simulink model "insulin_model"  (R2024b)
settings: Solver=ode15s  StartTime=0.0  StopTime=86400  MaxStep=0.5  RelTol=1e-3
libraries: fl_lib x11, nesl_utility x4, eeGeneralControl x1, SimscapeFluids_lib x1
settings Model: Creator=14083  LastModifiedBy=14083

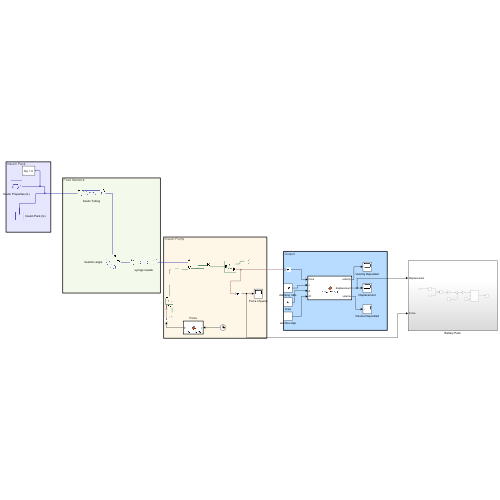
[thumbnail: Simulink's stored preview of the top-level diagram]
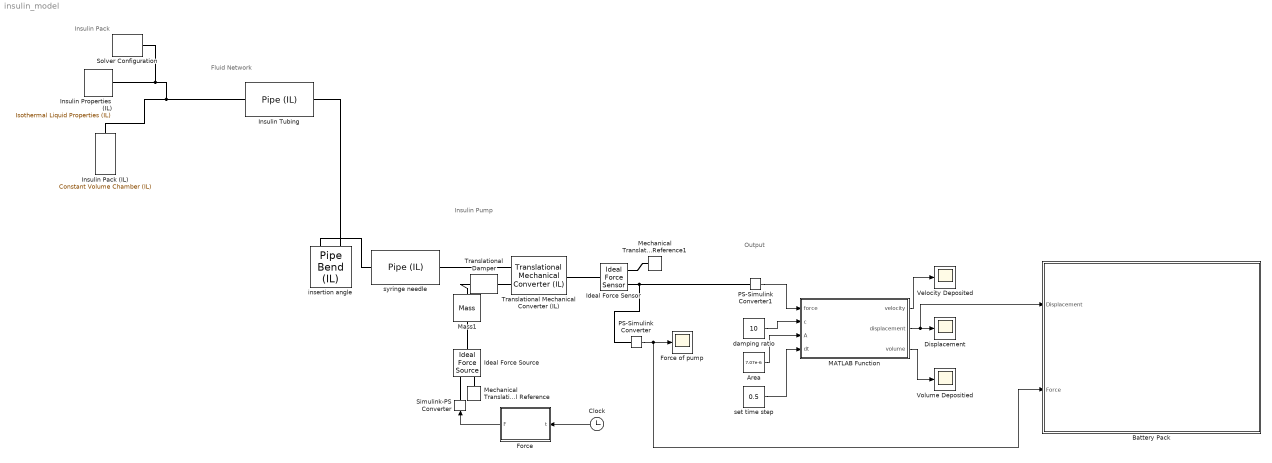
== system insulin_model ==
  note: Fluid Network
  note: Output
  note: Insulin Pump
  note: Insulin Pack
  Area : Constant  Value=7.07e-6
  Battery Pack : Subsystem
  Clock : Clock
  Displacement : Scope
  Force : MATLAB Function  TreatAsAtomicUnit=on
  Force of pump : Scope
  Ideal Force Sensor : fl_lib/Mechanical/Mechanical Sensors/Ideal Force Sensor
  Ideal Force Source : fl_lib/Mechanical/Mechanical Sources/Ideal Force Source
  Insulin Pack (IL) : fl_lib/Isothermal Liquid/Elements/Constant Volume Chamber (IL)  volume=0.00068 l  p_I_specify=off  p_I_priority=High  p_I=0.101325 MPa  p_I_nominal_specify=off  p_I_nominal_value=1  p_I_nominal_unit=MPa
      settings: InternalSimscapePortConfiguration="{\"Bottom\":[],\"Left\":[{\"id\":\"A\",\"label\":\"A\",\"type\":\"foundation.isothermal_liquid.isothermal_liquid\"}],\"Right\":[],\"Top\":[]}"
  Insulin Properties (IL) : fl_lib/Isothermal Liquid/Utilities/Isothermal Liquid Properties (IL)  rho_L_atm=998.2 kg/m^3  bulk_modulus_model=foundation.enum.bulk_modulus_model.const  beta_gain=6  beta_L_atm=2.1791e9 Pa  nu_atm=1.0034e-6 m^2/s  p_atm=0.101325 MPa  p_min=1 Pa  properties_range_check=simscape.enum.assert.action.error  air_fraction=0.005  polytropic_index=1.0  rho_g_atm=1.225 kg/m^3  air_dissolution_model=false  p_crit=3 MPa
  Insulin Tubing : fl_lib/Isothermal Liquid/Elements/Pipe (IL)  length=23 in  area=(1.5^2)*pi/4 mm^2  Dh=1.5 mm  length_add=1 m  roughness=15e-6 m  Re_lam=2000  Re_tur=4000  shape_factor=64  dynamic_compressibility=true  inertia=false  p0=0.101325 MPa  mdot0=0 kg/s
      settings: InternalSimscapePortConfiguration="{\"Bottom\":[],\"Left\":[{\"id\":\"A\",\"label\":\"A\",\"type\":\"foundation.isothermal_liquid.isothermal_liquid\"}],\"Right\":[{\"id\":\"B\",\"label\":\"B\",\"type\":\"foundation.isothermal_liquid.isothermal_liquid\"}],\"Top\":[]}"
  MATLAB Function : MATLAB Function  TreatAsAtomicUnit=on  SystemSampleTime=0.5
  Mass1 : fl_lib/Mechanical/Translational Elements/Mass  mass=0.01 kg  num_ports=foundation.enum.numPorts2.two  v_specify=off  v_priority=High  v=0 m/s  v_nominal_specify=off  v_nominal_value=1  v_nominal_unit=m/s  f_specify=off  f_priority=None  f=0 N  f_nominal_specify=off  f_nominal_value=1  f_nominal_unit=N
      settings: InternalSimscapePortConfiguration="{\"Bottom\":[],\"Left\":[{\"id\":\"M\",\"label\":\"\",\"type\":\"foundation.mechanical.translational.translational\"}],\"Right\":[{\"id\":\"N\",\"label\":\"\",\"type\":\"foundation.mechanical.translational.translational\"}],\"Top\":[]}"
  Mechanical Translational Reference : fl_lib/Mechanical/Translational Elements/Mechanical Translational Reference
  Mechanical Translational Reference1 : fl_lib/Mechanical/Translational Elements/Mechanical Translational Reference
  PS-Simulink Converter : nesl_utility/PS-Simulink Converter  PhysicalDomain=network_engine_domain  SubClassName=ps_output  LeftPortType=input  RightPortType=output  PseudoPeriodic=off  Frequencies=[]  VectorFormat=inherit  Unit=inherit  AffineConversion=off
  PS-Simulink Converter1 : nesl_utility/PS-Simulink Converter  PhysicalDomain=network_engine_domain  SubClassName=ps_output  LeftPortType=input  RightPortType=output  PseudoPeriodic=off  Frequencies=[]  VectorFormat=inherit  Unit=inherit  AffineConversion=off
  Simulink-PS Converter : nesl_utility/Simulink-PS Converter  PhysicalDomain=network_engine_domain  SubClassName=ps_input  LeftPortType=input  RightPortType=output  PseudoPeriodic=off  Frequencies=[]  NoiseDistribution=none  NoiseParameters=[]  Unit=1  AffineConversion=off  FilteringAndDerivatives=provide  SimscapeFilterOrder=1  InputFilterTimeConstant=0.001  UdotUserProvided=0
  Solver Configuration : nesl_utility/Solver Configuration  PhysicalDomain=network_engine_domain  SubClassName=solver  LeftPortType=input  RightPortType=generic  Tones=[]  Harmonics=[]  SimulateNoise=off  Profile=off  UseLocalSampling=off  EnableSwitchedLinearOptims=on  FrequencyDomain=off  UseCCode=off  RelTol=0.001  AbsTol=0.001  MinStep=1e-09  ToWorkspace=off  RevertToSquareIcSolve=off  NumHomotopyIterations=100  PhasorMode=off  PhasorModeNumHarmonics=1  ConsistencySolver=NEWTON_XTOL_AFTER_FTOL  IndexReductionMethod=DerivativeReplacement  DoDC=off  ResidualTolerance=1e-09  ConsistencyTolSource=GLOBAL  ConsistencyAbsTol=0.001  ConsistencyRelTol=0.001  ConsistencyTolFactor=0.001  UseLocalSolver=off  LocalSolverChoice=NE_BACKWARD_EULER_ADVANCER  ResolveIndetEquations=on  FunctionEvalNumThread=1  LocalSolverSampleTime=0.001  DoFixedCost=off  MaxNonlinIter=3  MaxModeIter=2  ComputeImpulses=off  ImpulseIterations=2  LinearAlgebra=auto  LinearAlgebraNumThread=0  EquationFormulation=NE_TIME_EF  DelaysMemoryBudget=1024  AutomaticFiltering=on  FilteringTimeConstant=0.001  PartitionStorageMethod=AS_NEEDED  PartitionMemoryBudget=1024  PartitionMethod=ROBUST  MultibodyUseLocalSolver=off  MultibodyLocalSolverChoice=ODE1  MultibodyLocalSolverSampleTime=0.001
  Translational Mechanical Converter (IL) : fl_lib/Isothermal Liquid/Elements/Translational Mechanical Converter (IL)  mech_orientation=foundation.enum.MechOrientationTranslational.Positive  displacement_spec=foundation.enum.DisplacementSpec.Calculate  x0=0 m  interface_area=7.07*10^-6 m^2  dead_volume=0.0001 m^3  pressure_spec=foundation.enum.pressure_spec.atmospheric  environment_pressure=0.101325 MPa  dynamic_compressibility=true  p0=0.101325 MPa
      settings: InternalSimscapePortConfiguration="{\"Bottom\":[],\"Left\":[{\"id\":\"A\",\"label\":\"A\",\"type\":\"foundation.isothermal_liquid.isothermal_liquid\"},{\"id\":\"C\",\"label\":\"C\",\"type\":\"foundation.mechanical.translational.translational\"}],\"Right\":[{\"id\":\"R\",\"label\":\"R\",\"type\":\"foundation.mechanical.translational.translational\"}],\"Top\":[]}"
  Translational Damper : fl_lib/Mechanical/Translational Elements/Translational Damper  D=100 N*s/m  v_specify=off  v_priority=None  v=0 m/s  v_nominal_specify=off  v_nominal_value=1  v_nominal_unit=m/s  f_specify=off  f_priority=None  f=0 N  f_nominal_specify=off  f_nominal_value=1  f_nominal_unit=N
  Velocity Deposited : Scope
  Volume Depositied : Scope
  damping ratio : Constant  Value=10
  insertion angle : SimscapeFluids_lib/Isothermal Liquid/Pipes & Fittings/Pipe Bend (IL)  diameter_bend=0.184 mm  bend_radius=0.04 mm  angle_bend=30 deg  roughness=0.0015 mm  dynamic_compressibility=false  p0=0.101325 MPa
      settings: InternalSimscapePortConfiguration="{\"Bottom\":[],\"Left\":[{\"id\":\"A\",\"label\":\"A\",\"type\":\"foundation.isothermal_liquid.isothermal_liquid\"}],\"Right\":[],\"Top\":[{\"id\":\"B\",\"label\":\"B\",\"type\":\"foundation.isothermal_liquid.isothermal_liquid\"}]}"
  set time step : Constant  Value=0.5
  syringe needle : fl_lib/Isothermal Liquid/Elements/Pipe (IL)  length=5 mm  area=(0.362^2-0.184^2)*pi/4 mm^2  Dh=0.184 mm  length_add=1 m  roughness=15e-6 m  Re_lam=2000  Re_tur=4000  shape_factor=64  dynamic_compressibility=true  inertia=false  p0=0.101325 MPa  mdot0=0 kg/s
      settings: InternalSimscapePortConfiguration="{\"Bottom\":[],\"Left\":[{\"id\":\"A\",\"label\":\"A\",\"type\":\"foundation.isothermal_liquid.isothermal_liquid\"}],\"Right\":[{\"id\":\"B\",\"label\":\"B\",\"type\":\"foundation.isothermal_liquid.isothermal_liquid\"}],\"Top\":[]}"
  wires:
  Force/1(F) -> Simulink-PS Converter/1
  Clock/1 -> Force/1(t)
  PS-Simulink Converter1/1 -> MATLAB Function/1(force)
  damping ratio/1 -> MATLAB Function/2(c)
  Area/1 -> MATLAB Function/3(A)
  MATLAB Function/3(volume) -> Volume Depositied/1
  MATLAB Function/2(displacement) -> Battery Pack/1(Displacement), Displacement/1
  MATLAB Function/1(velocity) -> Velocity Deposited/1
  set time step/1 -> MATLAB Function/4(dt)
  PS-Simulink Converter/1 -> Battery Pack/2(Force), Force of pump/1
  connections:
  Insulin Properties (IL)/RConn1 -- Solver Configuration/RConn1 -- Insulin Tubing/LConn1 -- Insulin Pack (IL)/LConn1
  Translational Damper/LConn1 -- Translational Mechanical Converter (IL)/LConn2
  Translational Damper/RConn1 -- Mass1/LConn1
  Ideal Force Source/LConn1 -- Mass1/RConn1
  Simulink-PS Converter/RConn1 -- Ideal Force Source/RConn1
  Mechanical Translational Reference/LConn1 -- Ideal Force Source/RConn2
  Ideal Force Sensor/LConn1 -- Translational Mechanical Converter (IL)/RConn1
  Ideal Force Sensor/RConn1 -- Mechanical Translational Reference1/LConn1
  PS-Simulink Converter/LConn1 -- PS-Simulink Converter1/LConn1 -- Ideal Force Sensor/RConn2
  Insulin Tubing/RConn1 -- insertion angle/LConn1
  syringe needle/LConn1 -- insertion angle/LConn2
  syringe needle/RConn1 -- Translational Mechanical Converter (IL)/LConn1

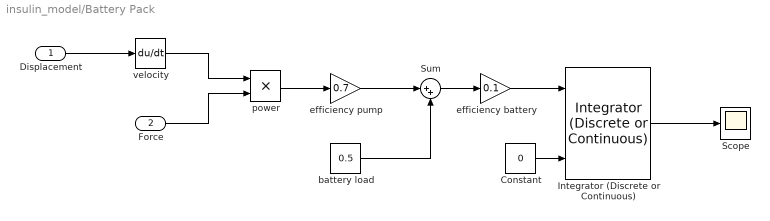
== system insulin_model/Battery Pack ==
  Displacement : Inport
  Force : Inport  Port=2
  Constant : Constant  Value=0
  Integrator (Discrete or Continuous) : eeGeneralControl/Integrator (Discrete or Continuous)  LabelModeActiveChoice=Discrete  ExternalReset=level  LimitType=Anti-windup  B=inf  A=-inf  Ts=0.5
      settings: LibrarySourceBlock=|
      | ee_sl_lib/General Control/Integrator
      | (Discrete or Continuous)
  Scope : Scope
  Sum : Sum  Inputs=|++
  battery load : Constant  Value=0.5
  efficiency battery : Gain  Gain=0.1
  efficiency pump : Gain  Gain=0.7
  power : Product
  velocity : Derivative
  wires:
  Displacement/1 -> velocity/1
  Force/1 -> power/2
  velocity/1 -> power/1
  power/1 -> efficiency pump/1
  battery load/1 -> Sum/2
  efficiency pump/1 -> Sum/1
  Sum/1 -> efficiency battery/1
  efficiency battery/1 -> Integrator (Discrete or Continuous)/1
  Constant/1 -> Integrator (Discrete or Continuous)/3
  Integrator (Discrete or Continuous)/1 -> Scope/1

== matlab function insulin_model/MATLAB Function ==
  data: force input; velocity output; c input; A input; displacement output; volume output; dt input
function [velocity, displacement, volume] = pistonModel(force, c, A, dt)

    persistent x
    if isempty(x)
        x = 0; 
    end

    if c == 0
        velocity = 0;
    else
        velocity = force / c;
    end

    x = x + velocity * dt;
    displacement = x;
    volume = A * x;
end

== matlab function insulin_model/Force ==
  data: t input; F output
function F = insulin_force(t)


force_per_unit = 0.35;      
pulse_duration = 15;       
F = 0;

if mod(t, 1800) < pulse_duration
    F = 0.5 * force_per_unit;
    return;
end

% injections at 8am, 12pm, 6pm, 10pm
times = [8, 12, 18, 22] * 3600;
doses = [12, 5, 20, 7];

for i = 1:length(times)
    if t >= times(i) && t < times(i) + pulse_duration
        F = doses(i) * force_per_unit;
        return;
    end
end

end
